simulink library "uavsimblockset_TrimKinematics"  (Simulink 8.0)
settings: Solver=ode45  StartTime=0.0  StopTime=10.0  RelTol=1e-3
undefined symbols (not defined in the file): Earth, WGS84
libraries: aerolib6dof2 x1, aerolibtransform2 x1, uavsimblockset_vbody2vNED x1
settings Model: Creator=mstolle  LastModifiedBy=j.bolting

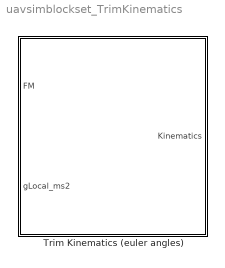
== system uavsimblockset_TrimKinematics ==
  Trim Kinematics (euler angles) : Subsystem  mask{mask_inertia=0, mask_mass=0, mask_P0_ECEF_m=0, mask_uvw0=0, mask_phithetapsi0=0, mask_omega0=0}
      mask prompts: mask_inertia "Inertia tensor [kg * m²]"; mask_mass "Aircraft mass [kg]"; mask_P0_ECEF_m "Initial ECEF position [m]"; mask_uvw0 "Initial velocity vector, body frame [m/s]"; mask_phithetapsi0 "Initial Euler angles [rad]"; mask_omega0 "Initial body rotation rates [rad/s]"

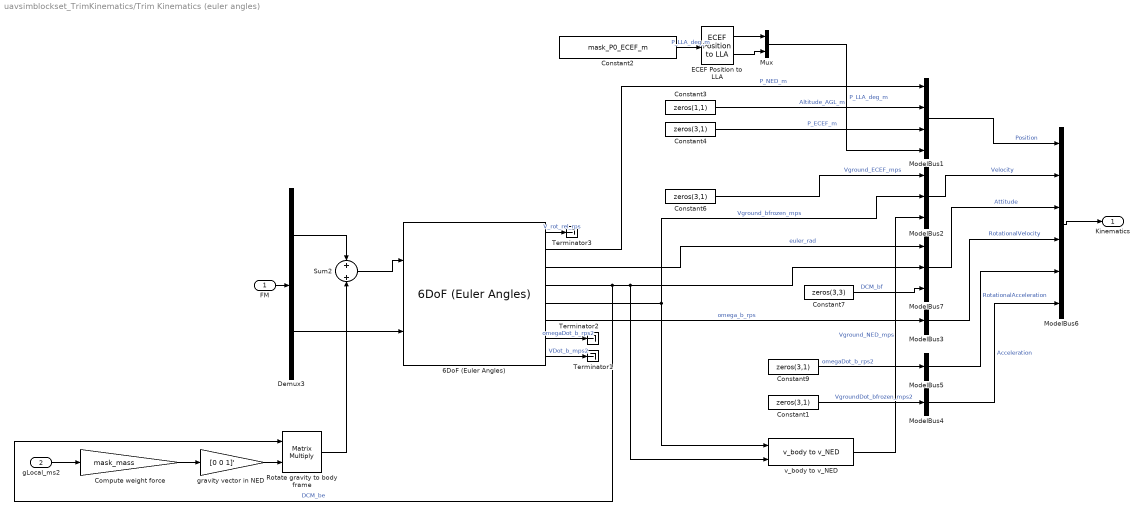
== system uavsimblockset_TrimKinematics/Trim Kinematics (euler angles) ==
  FM : Inport
  gLocal_ms2 : Inport  Port=2
  6DoF (Euler Angles) : aerolib6dof2/6DoF (Euler Angles)  units=Metric (MKS)  mtype=Fixed  rep=Euler Angles  xme_0=mask_P0_ECEF_m  Vm_0=mask_uvw0  eul_0=mask_phithetapsi0  pm_0=mask_omega0  mass_0=mask_mass  mass_e=0.5  mass_f=2.0  inertia=mask_inertia  inertia_e=eye(3)  inertia_f=2*eye(3)  k_quat=1.0
  Compute weight force : Gain  Gain=mask_mass
  Constant{1,4,6,9} (4 alike) : Constant  Value=zeros(3,1)
  Constant2 : Constant  Value=mask_P0_ECEF_m
  Constant3 : Constant  Value=zeros(1,1)
  Constant7 : Constant  Value=zeros(3,3)
  Demux3 : Demux  Outputs=[3,3]
  ECEF Position to LLA : aerolibtransform2/ECEF Position to LLA  units=Metric (MKS)  ptype=Earth (WGS84)  F=1/298.257223563  R=6378137
  ModelBus1 : BusCreator  Inputs='P_NED_m','Altitude_AGL_m','P_ECEF_m','P_LLA_deg_m'  OutDataTypeStr=Bus: Position  NonVirtualBus=on
  ModelBus2 : BusCreator  Inputs=3  OutDataTypeStr=Bus: Velocity  NonVirtualBus=on
  ModelBus3 : BusCreator  Inputs='omega_b_rps'  OutDataTypeStr=Bus: RotationalVelocity  NonVirtualBus=on
  ModelBus4 : BusCreator  Inputs=1  OutDataTypeStr=Bus: Acceleration  NonVirtualBus=on
  ModelBus5 : BusCreator  Inputs='omegaDot_b_rps2'  OutDataTypeStr=Bus: RotationalAcceleration  NonVirtualBus=on
  ModelBus6 : BusCreator  Inputs=6  OutDataTypeStr=Bus: Kinematics
  ModelBus7 : BusCreator  Inputs='euler_rad','DCM_be','DCM_bf'  OutDataTypeStr=Bus: Attitude  NonVirtualBus=on
  Mux : Mux  Inputs=2
  Rotate gravity to body frame : Product  Multiplication=Matrix(*)
  Sum2 : Sum  SaturateOnIntegerOverflow=on  InputSameDT=on  OutDataTypeStr=Inherit: Same as first input
  Terminator1 : Terminator
  Terminator2 : Terminator
  Terminator3 : Terminator
  gravity vector in NED : Gain  Gain=[0 0 1]'
  v_body to v_NED : uavsimblockset_vbody2vNED/v_body to v_NED
  Kinematics : Outport  OutDataTypeStr=Bus: Kinematics
  wires:
  ModelBus4/1 -> ModelBus6/6  "Acceleration"
  ModelBus1/1 -> ModelBus6/1  "Position"
  Constant4/1 -> ModelBus1/3  "P_ECEF_m"
  ModelBus7/1 -> ModelBus6/3  "Attitude"
  Demux3/1 -> Sum2/1
  6DoF (Euler Angles)/4 -> Rotate gravity to body frame/1, v_body to v_NED/2, ModelBus7/2  "DCM_be"
  6DoF (Euler Angles)/6 -> ModelBus3/1  "omega_b_rps"
  Sum2/1 -> 6DoF (Euler Angles)/1
  Demux3/2 -> 6DoF (Euler Angles)/2
  Constant6/1 -> ModelBus2/1  "Vground_ECEF_mps"
  6DoF (Euler Angles)/3 -> ModelBus7/1  "euler_rad"
  ModelBus3/1 -> ModelBus6/4  "RotationalVelocity"
  ModelBus2/1 -> ModelBus6/2  "Velocity"
  ModelBus5/1 -> ModelBus6/5  "RotationalAcceleration"
  Constant3/1 -> ModelBus1/2  "Altitude_AGL_m"
  Mux/1 -> ModelBus1/4  "P_LLA_deg_m"
  6DoF (Euler Angles)/2 -> ModelBus1/1  "P_NED_m"
  6DoF (Euler Angles)/5 -> ModelBus2/2, v_body to v_NED/1  "Vground_bfrozen_mps"
  ModelBus6/1 -> Kinematics/1
  Constant1/1 -> ModelBus4/1  "VgroundDot_bfrozen_mps2"
  6DoF (Euler Angles)/8 -> Terminator1/1  "VDot_b_mps2"
  6DoF (Euler Angles)/7 -> Terminator2/1  "omegaDot_b_rps2"
  Constant9/1 -> ModelBus5/1  "omegaDot_b_rps2"
  FM/1 -> Demux3/1
  6DoF (Euler Angles)/1 -> Terminator3/1  "V_rot_rel_rps"
  Constant7/1 -> ModelBus7/3  "DCM_bf"
  v_body to v_NED/1 -> ModelBus2/3  "Vground_NED_mps"
  gLocal_ms2/1 -> Compute weight force/1
  gravity vector in NED/1 -> Rotate gravity to body frame/2
  Compute weight force/1 -> gravity vector in NED/1
  Rotate gravity to body frame/1 -> Sum2/2
  Constant2/1 -> ECEF Position to LLA/1  "P_LLA_deg_m"
  ECEF Position to LLA/1 -> Mux/1
  ECEF Position to LLA/2 -> Mux/2
